simulink model "whirlybird_sim"  (Simulink 8.1)
settings: Solver=ode45  StartTime=0.0  StopTime=300  RelTol=1e-3
undefined symbols (not defined in the file or in its folder): P, whirlybird_controller
libraries: simulink x2
settings Model: Creator=Administrator  LastModifiedBy=jhl48
settings GRTTargetCC: CodeReplacementLibrary=None  CPPClassGenCompliant=on

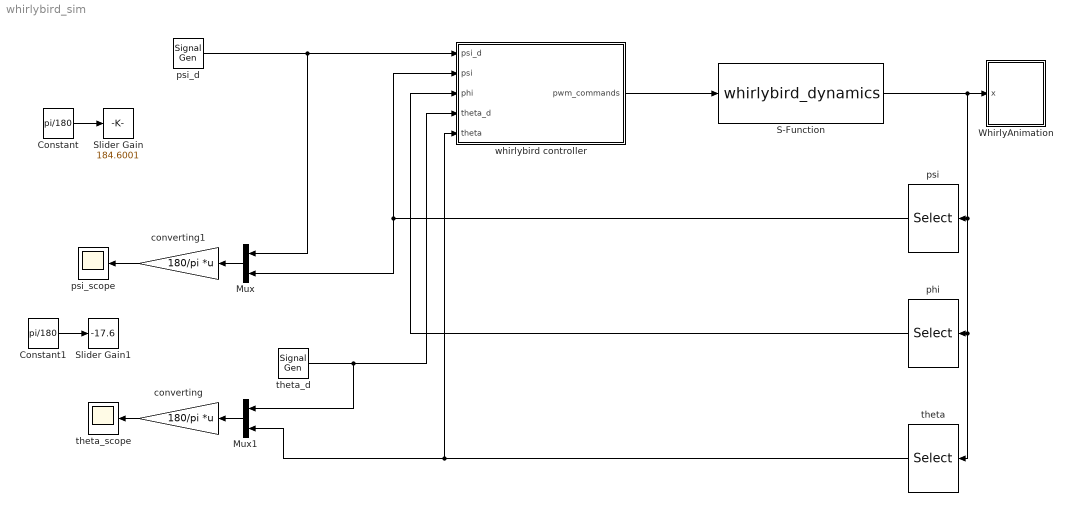
== system whirlybird_sim ==
  Constant : Constant  Value=pi/180
  Constant1 : Constant  Value=pi/180
  Mux : Mux  Inputs=2
  Mux1 : Mux  Inputs=2
  S-Function : S-Function  FunctionName=whirlybird_dynamics  Parameters=P  EnableBusSupport=off
  Slider Gain : simulink/Math Operations/Slider Gain  low=0  gain=184.6001  high=360
  Slider Gain1 : simulink/Math Operations/Slider Gain  low=-30  gain=-17.6  high=30
  WhirlyAnimation : Subsystem
      mask Display: image(imread('tv.jpg'))
  converting : Gain  Gain=180/pi  Multiplication=Matrix(K*u)
  converting1 : Gain  Gain=180/pi  Multiplication=Matrix(K*u)
  phi : Selector  InputPortWidth=6  IndexOptions=Index vector (dialog)  Indices=[1]  OutputSizes=1
  psi : Selector  InputPortWidth=6  IndexOptions=Index vector (dialog)  Indices=[5]  OutputSizes=1
  psi_d : SignalGenerator  WaveForm=square  Amplitude=60*pi/180  Frequency=0.1  Units=rad/sec
  psi_scope : Scope
      settings: YMin=-90  YMax=80
  theta : Selector  InputPortWidth=6  IndexOptions=Index vector (dialog)  Indices=[3]  OutputSizes=1
  theta_d : SignalGenerator  WaveForm=square  Amplitude=15*pi/180  Frequency=0.1  Units=rad/sec
  theta_scope : Scope
      settings: YMin=-25  YMax=25
  whirlybird controller : Subsystem
  wires:
  S-Function/1 -> psi/1, theta/1, phi/1, WhirlyAnimation/1(x)
  theta/1 -> whirlybird controller/5(theta), Mux1/2
  Mux1/1 -> converting/1
  converting/1 -> theta_scope/1
  converting1/1 -> psi_scope/1
  Mux/1 -> converting1/1
  psi/1 -> Mux/2, whirlybird controller/2(psi)
  whirlybird controller/1(pwm_commands) -> S-Function/1
  Constant/1 -> Slider Gain/1
  Constant1/1 -> Slider Gain1/1
  psi_d/1 -> Mux/1, whirlybird controller/1(psi_d)
  theta_d/1 -> Mux1/1, whirlybird controller/4(theta_d)
  phi/1 -> whirlybird controller/3(phi)

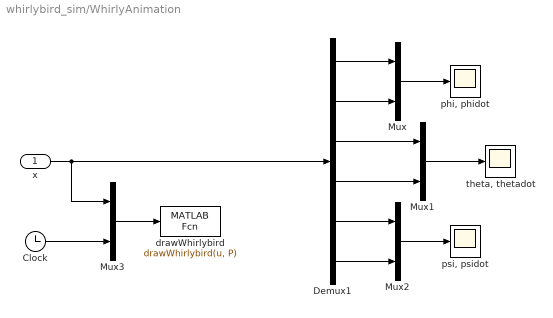
== system whirlybird_sim/WhirlyAnimation ==
  x : Inport
  Clock : Clock
  Demux1 : Demux  Outputs=6
  Mux{,1..3} (4 alike) : Mux  Inputs=2
  drawWhirlybird : MATLABFcn  MATLABFcn=drawWhirlybird(u, P)  OutputDimensions=0  SampleTime=0.1
  "phi, phidot" : Scope
      settings: TimeRange=40  YMin=-10  YMax=15  SaveName=ScopeData4
  "psi, psidot" : Scope
      settings: TimeRange=40  YMin=-2  YMax=1  SaveName=ScopeData3
  "theta, thetadot" : Scope
      settings: TimeRange=40  YMin=-2  YMax=1  SaveName=ScopeData2
  wires:
  Demux1/1 -> Mux/1
  Demux1/2 -> Mux/2
  Demux1/3 -> Mux1/1
  Demux1/4 -> Mux1/2
  Demux1/5 -> Mux2/1
  Demux1/6 -> Mux2/2
  Mux2/1 -> "psi, psidot"/1
  Mux1/1 -> "theta, thetadot"/1
  Mux/1 -> "phi, phidot"/1
  x/1 -> Mux3/1, Demux1/1
  Clock/1 -> Mux3/2
  Mux3/1 -> drawWhirlybird/1

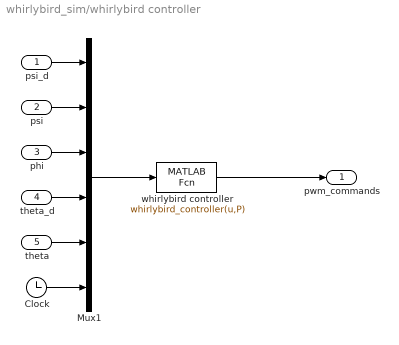
== system whirlybird_sim/whirlybird controller ==
  psi_d : Inport
  psi : Inport  Port=2
  phi : Inport  Port=3
  theta_d : Inport  Port=4
  theta : Inport  Port=5
  Clock : Clock
  Mux1 : Mux  Inputs=6
  whirlybird controller : MATLABFcn  MATLABFcn=whirlybird_controller(u,P)  OutputDimensions=2  SampleTime=P.Ts
  pwm_commands : Outport
  wires:
  Mux1/1 -> whirlybird controller/1
  psi_d/1 -> Mux1/1
  psi/1 -> Mux1/2
  whirlybird controller/1 -> pwm_commands/1
  phi/1 -> Mux1/3
  Clock/1 -> Mux1/6
  theta_d/1 -> Mux1/4
  theta/1 -> Mux1/5
